simulink model "plant_block"  (R2020b)
settings: Solver=ode1  StartTime=0.0  StopTime=300  RelTol=1e-3  EnableMultiTasking=on
undefined symbols (not defined in the file or in its folder): K3
libraries: pid_lib x2
settings Model: SimulationMode=external  Creator=Dro  LastModifiedBy=josh2
settings DataIOCC: LimitDataPoints=on  SaveFormat=Array  ReturnWorkspaceOutputs=off  SignalLoggingName=sigsOut
settings OptimizationCC: ExpressionDepthLimit=2147483647  InitFltsAndDblsToZero=on
settings DebuggingCC: SaveWithParameterizedLinksMsg=none  UnderspecifiedInitializationDetection=Classic  MergeDetectMultiDrivingBlocksExec=none  SignalResolutionControl=TryResolveAllWithWarning  MultiTaskDSMMsg=warning  MultiTaskCondExecSysMsg=none  FcnCallInpInsideContextMsg=warning  StateNameClashWarn=warning  SFUnexpectedBacktrackingDiag=warning  SFNoUnconditionalDefaultTransitionDiag=warning  SFExecutionAtInitializationDiag=none  ArithmeticOperatorsInVariantConditions=warning
settings HardwareCC: TargetBitPerLong=64  TargetBitPerPointer=64  TargetIntDivRoundTo=Zero  TargetEndianess=LittleEndian  TargetWordSize=64  TargetHWDeviceType=Intel->x86-64
settings ModelReferenceCC: PropagateSignalLabelsOutOfModel=off
settings SFSimCC: SimUseLocalCustomCode=off  CustomCodeUndefinedFunction=UseInterfaceOnly
settings RTWCC: Description=Simulink Desktop Real-Time  SystemTargetFile=sldrt.tlc  TemplateMakefile=sldrt.tmf  RTWUseLocalCustomCode=off  RTWCompilerOptimization=on
settings CodeAppCC: MaxIdLength=95  StateflowObjectComments=on
settings TargetCC: TargetPreCompLibLocation=C:\Program Files\MATLAB\R2019b\toolbox\sldrt\lib\win64  ModelReferenceCompliant=off  CompOptLevelCompliant=off
settings ConfigComp: CovMetricSettings=dw  CovSaveCumulativeToWorkspaceVar=on  CovSaveSingleToWorkspaceVar=on  CovExternalEMLEnable=off

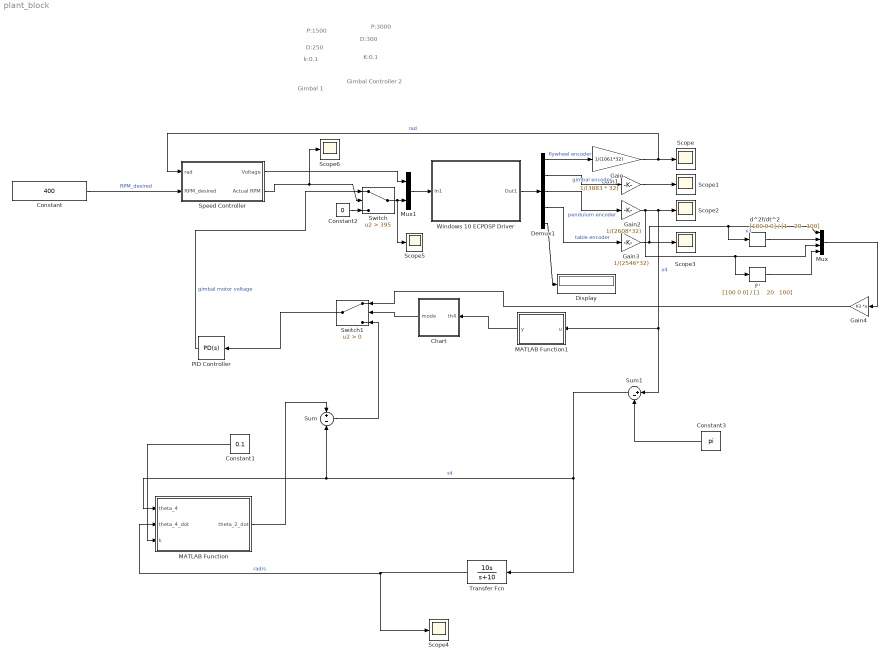
== system plant_block ==
  note: Gimbal Controller 2
  note: K:0.1
  note: D:300
  note: P:3000
  note: Gimbal 1
  note: k:0.1
  note: D:250
  note: P:1500
  Chart : Stateflow chart  TreatAsAtomicUnit=on
      settings: PortSchema="{\"entries\":[{\"content\":{\"sides\":[{\"content\":{\"connectorIds\":[\"Out1\"]},\"type\":\"ConnectorPlacement.EquallySpacedRectSide\",\"uuid\":\"9953b6da-b2d3-4ce5-b133-9611f64d20f4\"},{\"content\":{\"connectorIds\":[\"In1\"],\"side\":\"RIGHT\"},\"type\":\"ConnectorPlacement.EquallySpacedRectSide\",\"uuid\":\"e3288883-f4ff-49a0-9321-528b7a0e5843\"},{\"content\":{\"connectorIds\":[],\"side\":\"TOP\"},\"type\":\"ConnectorPlacement.EquallySpacedRectSide\",\"uuid\":\"97933b52-df16-4cb8-b063-db582d45748e\"},{\"content\":{\"connectorIds\":[],\"side\":\"HIDDEN\"},\"type\":\"ConnectorPlacement.EquallySpacedRectSide\",\"uuid\":\"7f48187c-aef4-4f80-a8fc-c0f4c8188bac\"}]},\"type\":\"ConnectorPlacement.EquallySpacedConnector\",\"uuid\":\"660afd19-2046-418b-8124-898d4ab32474\"}],\"packageUris\":[\"http://schema.mathworks.com/mf0/Connector/R2020b\"],\"version\":\"1.0\"}"
  Constant : Constant  Value=400
  Constant1 : Constant  Value=0.1
  Constant2 : Constant  Value=0
  Constant3 : Constant  Value=pi
  Demux1 : Demux  Outputs=5
      settings: DisplayOption=none
  Display : Display
  Gain : Gain  Gain=1/(1061*32)
  Gain1 : Gain  Gain=1/(3883 * 32)
  Gain2 : Gain  Gain=1/(2608*32)
  Gain3 : Gain  Gain=1/(2546*32)
  Gain4 : Gain  Gain=K3  Multiplication=Matrix(K*u)
  MATLAB Function : MATLAB Function  TreatAsAtomicUnit=on
  MATLAB Function1 : MATLAB Function  TreatAsAtomicUnit=on
  Mux : Mux
  Mux1 : Mux  Inputs=2
  PID Controller : pid_lib/PID Controller  Controller=PD  Form=Parallel  TimeDomain=Continuous-time  UseExternalTs=off  SampleTime=-1  IntegratorMethod=Forward Euler  FilterMethod=Forward Euler  ControllerParametersSource=internal  P=1500  I=0  D=38  UseFilter=on  N=100  TunerSelectOption=Transfer Function Based (PID Tuner App)  InitialConditionSource=internal  InitialConditionForIntegrator=0  InitialConditionForFilter=0  DifferentiatorICPrevScaledInput=0  ExternalReset=none  TrackingMode=off  Kt=1  LimitOutput=off  SatLimitsSource=internal  UpperSaturationLimit=inf  LowerSaturationLimit=-inf  LinearizeAsGain=on  AntiWindupMode=none  Kb=1  POutMin=[]  POutMax=[]  IOutMin=[]  IOutMax=[]  DOutMin=[]  DOutMax=[]  NOutMin=[]  NOutMax=[]  SumOutMin=[]  SumOutMax=[]  SaturationOutMin=[]  SaturationOutMax=[]  PParamMin=[]  PParamMax=[]  IParamMin=[]  IParamMax=[]  DParamMin=[]  DParamMax=[]  NParamMin=[]  NParamMax=[]  KbParamMin=[]  KbParamMax=[]  KtParamMin=[]  KtParamMax=[]  KbOutMin=[]  KbOutMax=[]  KtOutMin=[]  KtOutMax=[]  IntegratorOutMin=[]  IntegratorOutMax=[]  FilterOutMin=[]  FilterOutMax=[]  SumI1OutMin=[]  SumI1OutMax=[]  SumI2OutMin=[]  SumI2OutMax=[]  SumI3OutMin=[]  SumI3OutMax=[]  SumI4OutMin=[]  SumI4OutMax=[]  SumDOutMin=[]  SumDOutMax=[]  DifferentiatorOutMin=[]  DifferentiatorOutMax=[]  FilterDiffOutCoefMin=[]  FilterDiffOutCoefMax=[]  ReciprocalOutMin=[]  ReciprocalOutMax=[]  SumDenOutMin=[]  SumDenOutMax=[]  SumNumOutMin=[]  SumNumOutMax=[]  DivideOutMin=[]  DivideOutMax=[]  UdiffTsProdOutMin=[]  UdiffTsProdOutMax=[]  NTsProdOutMin=[]  NTsProdOutMax=[]  UintegralTsProdOutMin=[]  UintegralTsProdOutMax=[]  UngainTsProdOutMin=[]  UngainTsProdOutMax=[]  IntegratorContinuousStateAttributes=''  IntegratorStateMustResolveToSignalObject=off  IntegratorRTWStateStorageClass=Auto  FilterContinuousStateAttributes=''  FilterStateMustResolveToSignalObject=off  FilterRTWStateStorageClass=Auto  ParallelPVariant=InternalParameters  IdealPVariant=Disabled  IVariant=Disabled  DVariant=InternalParameters  IntegratorVariant=Disabled  SatVariant=Disabled  AWVariant=Disabled  PCopyVariant=Disabled  TRVariant=Disabled  FdbkBlocksVariant=Forward  IdealPFdbkVariant=Disabled  SatFdbkVariant=Disabled  DerivativeFilterVariant=ContFilter  NVariant=InternalParameters  NCopyVariant=Disabled  FilterICVariant=InternalICsFilter  IntegratorICVariant=Disabled  ExternalResetVariant=Disabled  TRSumVariant=Passthrough  SumFdbkVariant=Disabled  SumVariant=Sum_PD  TsampFilterVariant=InternalTs  TsampNgainVariant=Passthrough  TsampIntegralVariant=Disabled_SignalSpec  ExternalSaturationOutDataTypeStr=Inherit: Same as second input
  Scope{,1..6} (7 alike) : Scope
  "Speed Controller " : Subsystem
  Sum : Sum  Inputs=+-
  Sum1 : Sum  Inputs=|+-
  Switch : Switch  Criteria=u2 > Threshold  Threshold=395
  Switch1 : Switch  Criteria=u2 > Threshold
  Transfer Fcn : TransferFcn  Numerator=[10 0 ]  Denominator=[1 10]
  Windows 10 ECPDSP Driver : Subsystem  mask{BaseAddr='0x3F00', STime=0.008, TimeOutPer=500, HWAccess=on}
      mask prompts: BaseAddr "Base I/O Address"; STime "Sample Time (Sec)"; TimeOutPer "Timeout Period (500 ~ 2000)"; HWAccess "Hardware Access"
      mask Display: color('black');disp('ECPDSP Driver\n upto\n 4 Encs(ADC Channels)\n and 2 Dacs')
  d^2f/dt^2 : TransferFcn  Numerator=[100 0 0]  Denominator="[1    20   100]"
  f'' : TransferFcn  Numerator=[100 0 0]  Denominator="[1    20   100]"
  wires:
  Mux1/1 -> Windows 10 ECPDSP Driver/1(In1)
  Demux1/1 -> Gain/1  "flywheel encoder"
  Demux1/2 -> Gain1/1  "gimbal encoder"
  Demux1/3 -> Gain2/1  "pendulum encoder"
  Demux1/4 -> Gain3/1  "table encoder"
  PID Controller/1 -> Switch/1  "gimbal motor voltage"
  Windows 10 ECPDSP Driver/1(Out1) -> Demux1/1
  Demux1/5 -> Display/1
  Gain/1 -> "Speed Controller "/1(rad), Scope/1  "rad"
  Gain1/1 -> Scope1/1
  Gain3/1 -> Mux/1, d^2f/dt^2/1, Scope3/1  "x3"
  Constant/1 -> "Speed Controller "/2(RPM_desired)  "RPM_desired"
  "Speed Controller "/1(Voltage) -> Mux1/1
  Transfer Fcn/1 -> Scope4/1, MATLAB Function/2(theta_4_dot)  "rad/s"
  MATLAB Function/1(theta_2_dot) -> Sum/1
  Switch1/1 -> PID Controller/1
  Constant1/1 -> MATLAB Function/3(k)
  "Speed Controller "/2("Actual RPM ") -> Scope6/1, Switch/2
  Switch/1 -> Scope5/1, Mux1/2
  Constant2/1 -> Switch/3
  Constant3/1 -> Sum1/2
  Sum1/1 -> Sum/2, MATLAB Function/1(theta_4), Transfer Fcn/1  "t4"
  Gain2/1 -> f''/1, Mux/3, Scope2/1, Sum1/1, MATLAB Function1/1(u)  "x4"
  Mux/1 -> Gain4/1
  d^2f/dt^2/1 -> Mux/2
  f''/1 -> Mux/4
  Gain4/1 -> Switch1/1
  Chart/1(mode) -> Switch1/2
  Sum/1 -> Switch1/3
  MATLAB Function1/1(y) -> Chart/1(th4)

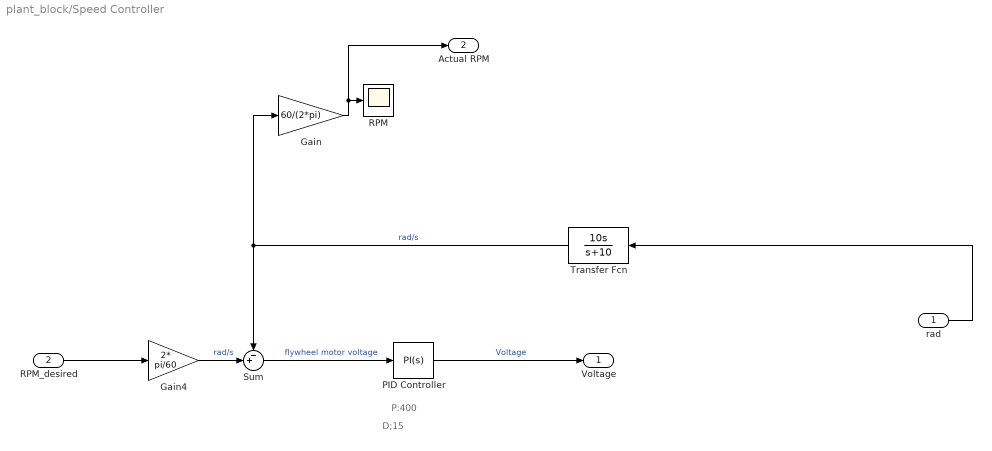
== system plant_block/Speed Controller  ==
  note: D;15
  note: P:400
  rad : Inport
  RPM_desired : Inport  Port=2
  Gain : Gain  Gain=60/(2*pi)
  Gain4 : Gain  Gain=2* pi/60
  PID Controller : pid_lib/PID Controller  Controller=PI  Form=Parallel  TimeDomain=Continuous-time  UseExternalTs=off  SampleTime=-1  IntegratorMethod=Forward Euler  FilterMethod=Forward Euler  ControllerParametersSource=internal  P=400  I=15  D=0  UseFilter=on  N=100  TunerSelectOption=Transfer Function Based (PID Tuner App)  InitialConditionSource=internal  InitialConditionForIntegrator=0  InitialConditionForFilter=0  DifferentiatorICPrevScaledInput=0  ExternalReset=none  TrackingMode=off  Kt=1  LimitOutput=off  SatLimitsSource=internal  UpperSaturationLimit=inf  LowerSaturationLimit=-inf  LinearizeAsGain=on  AntiWindupMode=none  Kb=1  POutMin=[]  POutMax=[]  IOutMin=[]  IOutMax=[]  DOutMin=[]  DOutMax=[]  NOutMin=[]  NOutMax=[]  SumOutMin=[]  SumOutMax=[]  SaturationOutMin=[]  SaturationOutMax=[]  PParamMin=[]  PParamMax=[]  IParamMin=[]  IParamMax=[]  DParamMin=[]  DParamMax=[]  NParamMin=[]  NParamMax=[]  KbParamMin=[]  KbParamMax=[]  KtParamMin=[]  KtParamMax=[]  KbOutMin=[]  KbOutMax=[]  KtOutMin=[]  KtOutMax=[]  IntegratorOutMin=[]  IntegratorOutMax=[]  FilterOutMin=[]  FilterOutMax=[]  SumI1OutMin=[]  SumI1OutMax=[]  SumI2OutMin=[]  SumI2OutMax=[]  SumI3OutMin=[]  SumI3OutMax=[]  SumI4OutMin=[]  SumI4OutMax=[]  SumDOutMin=[]  SumDOutMax=[]  DifferentiatorOutMin=[]  DifferentiatorOutMax=[]  FilterDiffOutCoefMin=[]  FilterDiffOutCoefMax=[]  ReciprocalOutMin=[]  ReciprocalOutMax=[]  SumDenOutMin=[]  SumDenOutMax=[]  SumNumOutMin=[]  SumNumOutMax=[]  DivideOutMin=[]  DivideOutMax=[]  UdiffTsProdOutMin=[]  UdiffTsProdOutMax=[]  NTsProdOutMin=[]  NTsProdOutMax=[]  UintegralTsProdOutMin=[]  UintegralTsProdOutMax=[]  UngainTsProdOutMin=[]  UngainTsProdOutMax=[]  IntegratorContinuousStateAttributes=''  IntegratorStateMustResolveToSignalObject=off  IntegratorRTWStateStorageClass=Auto  FilterContinuousStateAttributes=''  FilterStateMustResolveToSignalObject=off  FilterRTWStateStorageClass=Auto  ParallelPVariant=InternalParameters  IdealPVariant=Disabled  IVariant=InternalParameters  DVariant=Disabled  IntegratorVariant=Continuous  SatVariant=Disabled  AWVariant=Passthrough  PCopyVariant=Disabled  TRVariant=Disabled  FdbkBlocksVariant=Forward  IdealPFdbkVariant=Disabled  SatFdbkVariant=Disabled  DerivativeFilterVariant=Disabled  NVariant=Disabled  NCopyVariant=Disabled_SignalSpec  FilterICVariant=Disabled  IntegratorICVariant=InternalICs  ExternalResetVariant=Disabled  TRSumVariant=Passthrough  SumFdbkVariant=Disabled  SumVariant=Sum_PI  TsampFilterVariant=InternalTs  TsampNgainVariant=Passthrough  TsampIntegralVariant=Passthrough  ExternalSaturationOutDataTypeStr=Inherit: Same as second input
  RPM : Scope
  Sum : Sum  Inputs=-+|
  Transfer Fcn : TransferFcn  Numerator=[10 0 ]  Denominator=[1 10]
  Voltage : Outport
  "Actual RPM " : Outport  Port=2
  wires:
  Gain4/1 -> Sum/2  "rad/s"
  Transfer Fcn/1 -> Gain/1, Sum/1  "rad/s"
  Sum/1 -> PID Controller/1  "flywheel motor voltage"
  PID Controller/1 -> Voltage/1  "Voltage"
  RPM_desired/1 -> Gain4/1
  rad/1 -> Transfer Fcn/1
  Gain/1 -> "Actual RPM "/1, RPM/1

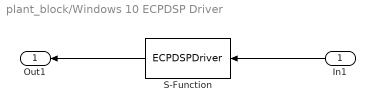
== system plant_block/Windows 10 ECPDSP Driver ==
  In1 : Inport
  S-Function : S-Function  FunctionName=ECPDSPDriver  Parameters=BaseAddr,STime,TimeOutPer,HWAccess  SFunctionDeploymentMode=off  EnableBusSupport=off
  Out1 : Outport
  wires:
  In1/1 -> S-Function/1
  S-Function/1 -> Out1/1

== matlab function plant_block/MATLAB Function1 ==
  data: u input; y output
function y = fcn(u)
% Returns the maximum difference between angular maxima
y = max(abs(mod(u, 2*pi)), abs(mod(u, 2*pi) - 2 * pi));

== matlab function plant_block/MATLAB Function ==
  data: theta_4 input; theta_2_dot output; theta_4_dot input; k input
function theta_2_dot = fcn(theta_4, theta_4_dot, k)

theta_2_dot = -(36353776222982492160*k*theta_4_dot*cos(theta_4)*((3314449799178915*theta_4_dot^2)/576460752303423488 + (7532743254738029*cos(theta_4))/18014398509481984 - 7532743254738029/18014398509481984))/(299580375726665093*pi);

end

== stateflow chart plant_block/Chart ==
  state CaptureController
    entry:
    mode=1
  state SwingUp
    entry:
    mode=0
  (default) -> SwingUp
  SwingUp -> CaptureController
  CaptureController -> SwingUp
  data: th4 input; mode output
